simulink model "ServoController"  (R2020a)
settings: Solver=ode3  StartTime=0.0  StopTime=inf  FixedStep=1/30  RelTol=1e-3  EnableMultiTasking=on
libraries: arduinolib x4
settings Model: FPTRunName=Active  SILPILModeSetting=veronly  ExtModeTrigDuration=2  Creator=The MathWorks, Inc.  LastModifiedBy=vince
settings DataIOCC: LimitDataPoints=on  SaveFormat=Array  ReturnWorkspaceOutputs=off
settings OptimizationCC: ExpressionDepthLimit=2147483647  LifeSpan=Inf  MaxStackSize=64
settings DebuggingCC: UnderspecifiedInitializationDetection=Classic  MergeDetectMultiDrivingBlocksExec=none  FcnCallInpInsideContextMsg=warning  AllowSymbolicDim=off  StateNameClashWarn=warning  SFUnexpectedBacktrackingDiag=warning  SFNoUnconditionalDefaultTransitionDiag=warning  SFExecutionAtInitializationDiag=none  ArithmeticOperatorsInVariantConditions=warning
settings HardwareCC: ProdBitPerInt=16  ProdBitPerPointer=16  ProdBitPerSizeT=16  ProdBitPerPtrDiffT=16  ProdLargestAtomicFloat=None  ProdWordSize=8  ProdHWDeviceType=Atmel->AVR
settings ModelReferenceCC: PropagateSignalLabelsOutOfModel=off
settings SFSimCC: SimUseLocalCustomCode=off  MATLABDynamicMemAlloc=off
settings RTWCC: SystemTargetFile=ert.tlc  HardwareBoard=Arduino Uno  TemplateMakefile=ert_default_tmf  GenerateReport=on  RTWVerbose=off  RTWUseLocalCustomCode=off  Toolchain=Arduino AVR  BuildConfiguration=Faster Runs  LaunchReport=on
settings CodeAppCC: ForceParamTrailComments=on  OperatorAnnotations=on  StateflowObjectComments=on  MATLABSourceComments=on
settings ERTTargetCC: MultiwordLength=2048  ERTCustomFileBanners=off  SupportContinuousTime=on  SupportNonInlinedSFcns=on  RemoveResetFunc=off  SupportVariableSizeSignals=on  ModelStepFunctionPrototypeControlCompliant=off  ExtModeStaticAllocSize=250
settings ConfigComp: CovMetricSettings=dw  CovHtmlReporting=on  CovSaveCumulativeToWorkspaceVar=on  CovSaveSingleToWorkspaceVar=on  CovExternalEMLEnable=off  CovSFcnEnable=off

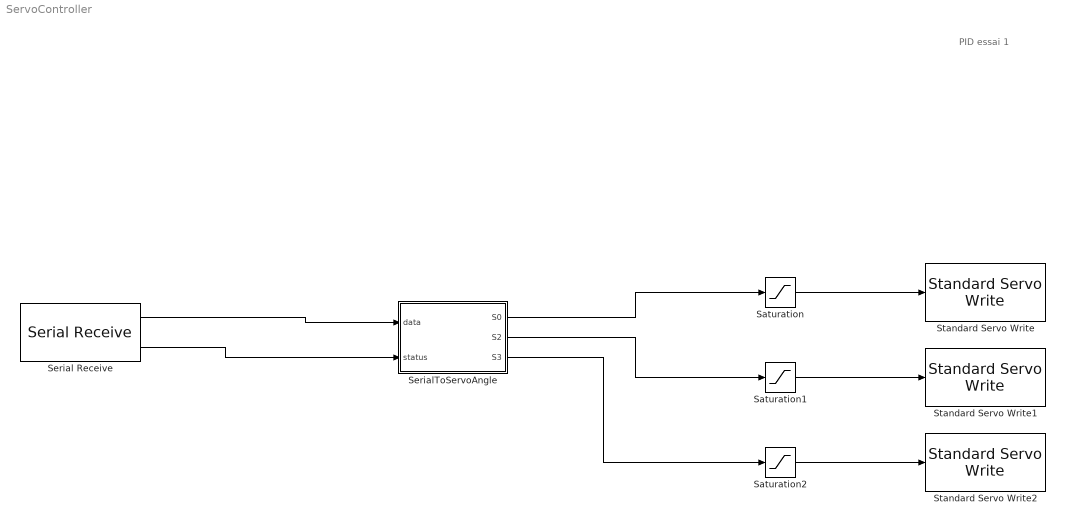
== system ServoController ==
  note: PID essai 1
  Saturation : Saturate  UpperLimit=35  LowerLimit=0
  Saturation1 : Saturate  UpperLimit=35  LowerLimit=0
  Saturation2 : Saturate  UpperLimit=35  LowerLimit=0
  Serial Receive : arduinolib/Serial Receive  isARMArch=off  portNumber=0  DataType=double  Datalength=3  SampleTime=0.2  showOutStatus=on  blockPlatform=arduino
      settings: SourceProductBaseCode=ARDUINO
  SerialToServoAngle : MATLAB Function  TreatAsAtomicUnit=on
  Standard Servo Write : arduinolib/Standard Servo Write  pinNumber=3  ServoIndex=0  blockPlatform=ARDUINO
  Standard Servo Write1 : arduinolib/Standard Servo Write  pinNumber=4  ServoIndex=1  blockPlatform=ARDUINO
  Standard Servo Write2 : arduinolib/Standard Servo Write  pinNumber=5  ServoIndex=2  blockPlatform=ARDUINO
  wires:
  Saturation/1 -> Standard Servo Write/1
  Saturation2/1 -> Standard Servo Write2/1
  Saturation1/1 -> Standard Servo Write1/1
  Serial Receive/2 -> SerialToServoAngle/2(status)
  Serial Receive/1 -> SerialToServoAngle/1(data)
  SerialToServoAngle/2(S2) -> Saturation1/1
  SerialToServoAngle/1(S0) -> Saturation/1
  SerialToServoAngle/3(S3) -> Saturation2/1

== matlab function ServoController/SerialToServoAngle ==
  data: S0 output double size=[1]; data input double size=[3]; S2 output double size=[1]; S3 output double size=[1]; status input
function [S0,S2, S3]  = SerialToServoAngle(data, status)
if(status==0)
    S0=0;
    S2=0;
    S3=0;
else
S0=data(1);
S2=data(2);
S3=data(3);
end
